simulink library "lib_transmission2"  (Simulink 4.1.1)
values from neighbouring files (symbols this model uses):
  logFlag = 1    [advSACompMaskInit.m]    (also in advSACompMaskInitR13.m)
undefined symbols (not defined in the file or in its folder): cyc_mph, fc_map_spd, fc_max_trq, fc_spd_scale, fc_trq_scale, fd_inertia, fd_loss, fd_ratio, gb_dnshift_load, gb_dnshift_spd, gb_gear_number_lookup, gb_gears_num, gb_inertia, gb_loss_const, gb_loss_input_spd_coeff, gb_loss_input_trq_coeff, gb_loss_output_spd_coeff, gb_loss_output_trq_coeff, gb_map_spd_out, gb_map_trq_in, gb_map_trq_out, gb_num_init, gb_ratio, gb_shift_delay, gb_spd_scale, gb_trq_scale, gb_upshift_load, gb_upshift_spd, htc_inertia, htc_k_adv, htc_k_adv_coast, htc_lockup, htc_lockup_load, htc_lockup_spd, htc_lu_gear_range, htc_max_coast_tr, htc_min_coast_tr, htc_pump_loss_spd, htc_pump_loss_trq_lockup, htc_pump_loss_trq_unlock, htc_sr, htc_sr_coast, htc_tr, htc_tr_coast, htc_unlock_spd, mc_map_spd, mc_max_trq, mc_overtrq_factor, mc_spd_scale, mc_trq_scale, tc_loss, tc_mc_to_fc_ratio, tx_eff_map, tx_map_spd, tx_map_trq, tx_pg_r, tx_pg_s, tx_speed_dep, vc_clutch_bool, vc_idle_spd ... (+2)
libraries: lib_controls x1, lib_etc x1, lib_controls2 x1, lib_transmission x1
(part 15 of 17)

== system lib_transmission2/hydraulic torque converter <htc> with pump loss/conventional HTC  and Interface/htc model/SR ==
  T,w req out : Inport  Port=1  LatchInput=off
  w in : Inport  Port=2  LatchInput=off
  >0 : Saturate  UpperLimit=inf  LowerLimit=eps  LinearizeAsGain=on
  Constant : Constant  Orientation=left  Value=0
  Constant1 : Constant  Value=vc_idle_spd+eps
  Constant3 : Constant  Value=1
  K_adv : Subsystem
      settings: RTWFcnNameOpts=Auto  RTWFileNameOpts=Auto
  K_adv_coast : Subsystem
      settings: RTWFcnNameOpts=Auto  RTWFileNameOpts=Auto
  Logical Operator : Logic  Operator=NOT  Inputs=1
  Logical Operator1 : Logic  Operator=NOT  Inputs=1
  MinMax : MinMax  Function=min  Inputs=2
  Relational Operator : RelationalOperator  Operator=>=
  SR Look-Up Table SR=wout/win : Lookup  InputValues=htc_k_adv  OutputValues=htc_sr
  SR Look-Up Table SR=wout/win coast : Lookup  InputValues=fliplr(htc_k_adv_coast)  OutputValues=fliplr(htc_sr_coast)
  SRmax= wout/win,min : Product  Inputs=*/  Multiplication=Element-wise(.*)  SaturateOnIntegerOverflow=on
  T : Selector  InputType=Vector  ElementSrc=Internal  Elements=1  RowSrc=Internal  Rows=1  ColumnSrc=Internal  Columns=1  InputPortWidth=2
  enhancedToWorkspace1 : Subsystem  TreatAsAtomicUnit=on  mask(enhancedToWorkspace){generalName=generalName, specificName=coasting, logFlag=logFlag}
      mask prompts: generalName "General Name [char-evaluated]"; specificName "Specific Name [char-literal]"; logFlag "Enable flag (1=on,0=off)"
      mask help: A wrapper for the Simulink "To Workspace" block that allows you to evaluate the name of the variable to log to workspace. This is useful to avoid the double logging errors that occur when you pull in two library models that attempt to log to the same variable.
      mask init:
      | enhancedToWsMaker
      settings: CopyFcn=breakLinkCopyFcn  ParentCloseFcn=breakLinkParCloseFcn  RTWFcnNameOpts=Auto  RTWFileNameOpts=Auto
      mask Help:
      | <h2>Enhanced To Workspace Block</h2>
      | <h3>Parameters</h3>
      | <UL>
      | <li><b>General Name:</b> This is the more general name of the variable. Variables are saved to the workspace as <i>generalName_specificName</i>. Note that this is an evaluated variable. If you would like to type in the value directly, it must be surrounded with single quotes. Otherwise you can input the name of a variable containing a char string.</li>
      | <li><b>Specific Name:</b> This is the specific name of the variable. Note that this is input as a char literal (i.e., you don't need quotes).</li>
      | <li><b>Enable Flag:</b> This flag should have the value of 0 or 1. If 0, the variable will not be logged to the workspace. If 1, the variable will be logged. This is done so that variable logging can be turned off to improve speed.</li>
      | </ul>
      | <h3>Overview</h3>
      | <p>The enhanced to workspace block was put together to allow one to dynamically resolve variable names at run time in simulink. This is most powerful when used in conjunction with a masked subsystem to allow multiple instances of that masked subsytem to be used in the same model. The strategy is to set the generalName in the block mask which will allow the block to change the general name for all variable logging on the fly.
      | <h3>Helper Files</h3>
      | <p>Three m-files are required by the enhancedToWorkspace block. These files are located in the &lt; ADVISOR root &gt;/GUI directory :
      | <ul>
      | <li><i>enhancedToWsMaker.m</i> This file runs the mask initialization for the block</li>
      | <li><i>breakLinkCopyFcn.m</i> This file is used by the block callback when the simulink block is copied. It is necessary to break the link to the enhancedToWorkspace similar to the To Workspace block in order for it to be able to configure itself. (Try copying simulink's To Workspace block--it is impossible to make a link)</li>
      | <li><i>breakLinkParCloseFcn.m</i> This file is similar to the breakLinkCopyFcn and is used when a parent system is closed</li>
      | </ul>
      | <hr>
      | 
      | <p>Created 2003-Jan-21, Michael Patrick O'Keefe, NREL</p>
      | 
      | <!--
      | <VARDEF>
      | <H3>var_name</H3>
      | <UL>
      | <LI><B>data type</B> data type here</LI>
      | <LI><B>units</B> units here</LI>
      | <LI><B>vehicle type</B> vehicle type here</LI>
      | <LI><B>description</B> description here</LI>
      | </UL>
      | </VARDEF>
      | -->
      mask Display: disp([generalName,'_',specificName])
  enhancedToWorkspace2 : Subsystem  TreatAsAtomicUnit=on  mask(enhancedToWorkspace){generalName=generalName, specificName=locked, logFlag=logFlag}
      mask prompts: generalName "General Name [char-evaluated]"; specificName "Specific Name [char-literal]"; logFlag "Enable flag (1=on,0=off)"
      mask help: A wrapper for the Simulink "To Workspace" block that allows you to evaluate the name of the variable to log to workspace. This is useful to avoid the double logging errors that occur when you pull in two library models that attempt to log to the same variable.
      mask init:
      | enhancedToWsMaker
      settings: CopyFcn=breakLinkCopyFcn  ParentCloseFcn=breakLinkParCloseFcn  RTWFcnNameOpts=Auto  RTWFileNameOpts=Auto
      mask Help:
      | <h2>Enhanced To Workspace Block</h2>
      | <h3>Parameters</h3>
      | <UL>
      | <li><b>General Name:</b> This is the more general name of the variable. Variables are saved to the workspace as <i>generalName_specificName</i>. Note that this is an evaluated variable. If you would like to type in the value directly, it must be surrounded with single quotes. Otherwise you can input the name of a variable containing a char string.</li>
      | <li><b>Specific Name:</b> This is the specific name of the variable. Note that this is input as a char literal (i.e., you don't need quotes).</li>
      | <li><b>Enable Flag:</b> This flag should have the value of 0 or 1. If 0, the variable will not be logged to the workspace. If 1, the variable will be logged. This is done so that variable logging can be turned off to improve speed.</li>
      | </ul>
      | <h3>Overview</h3>
      | <p>The enhanced to workspace block was put together to allow one to dynamically resolve variable names at run time in simulink. This is most powerful when used in conjunction with a masked subsystem to allow multiple instances of that masked subsytem to be used in the same model. The strategy is to set the generalName in the block mask which will allow the block to change the general name for all variable logging on the fly.
      | <h3>Helper Files</h3>
      | <p>Three m-files are required by the enhancedToWorkspace block. These files are located in the &lt; ADVISOR root &gt;/GUI directory :
      | <ul>
      | <li><i>enhancedToWsMaker.m</i> This file runs the mask initialization for the block</li>
      | <li><i>breakLinkCopyFcn.m</i> This file is used by the block callback when the simulink block is copied. It is necessary to break the link to the enhancedToWorkspace similar to the To Workspace block in order for it to be able to configure itself. (Try copying simulink's To Workspace block--it is impossible to make a link)</li>
      | <li><i>breakLinkParCloseFcn.m</i> This file is similar to the breakLinkCopyFcn and is used when a parent system is closed</li>
      | </ul>
      | <hr>
      | 
      | <p>Created 2003-Jan-21, Michael Patrick O'Keefe, NREL</p>
      | 
      | <!--
      | <VARDEF>
      | <H3>var_name</H3>
      | <UL>
      | <LI><B>data type</B> data type here</LI>
      | <LI><B>units</B> units here</LI>
      | <LI><B>vehicle type</B> vehicle type here</LI>
      | <LI><B>description</B> description here</LI>
      | </UL>
      | </VARDEF>
      | -->
      mask Display: disp([generalName,'_',specificName])
  if coasting : Switch  Threshold=eps
  "locked up, then SR=1" : Switch  Threshold=eps
  min,max : Saturate  UpperLimit=inf  LowerLimit=1  LinearizeAsGain=on
  shifting SR : Subsystem
      settings: RTWFcnNameOpts=Auto  RTWFileNameOpts=Auto
  wout,req : Selector  InputType=Vector  ElementSrc=Internal  Elements=2  RowSrc=Internal  Rows=1  ColumnSrc=Internal  Columns=1  InputPortWidth=2
  SR : Outport  Port=1  InitialOutput=0
  coasting : Outport  Port=2  InitialOutput=0
  wires:
  K_adv/1(K_adv) -> SR Look-Up Table SR=wout/win/1
  Logical Operator1/1 -> coasting/1, enhancedToWorkspace1/1(In1)
  >0/1 -> SR/1
  if coasting/1 -> >0/1
  K_adv_coast/1(K_adv_coast) -> SR Look-Up Table SR=wout/win coast/1
  MinMax/1 -> if coasting/3
  min,max/1 -> MinMax/1
  wout,req/1 -> SRmax= wout/win,min/1
  Constant1/1 -> SRmax= wout/win,min/2
  SRmax= wout/win,min/1 -> MinMax/2
  shifting SR/1(SR limited) -> if coasting/1
  "locked up, then SR=1"/1 -> shifting SR/3(SR)
  w in/1 -> shifting SR/2(w in)
  SR Look-Up Table SR=wout/win/1 -> "locked up, then SR=1"/1
  Constant3/1 -> "locked up, then SR=1"/3
  Logical Operator/1 -> "locked up, then SR=1"/2
  Relational Operator/1 -> Logical Operator1/1, if coasting/2
  T/1 -> Relational Operator/1
  Constant/1 -> Relational Operator/2
  SR Look-Up Table SR=wout/win coast/1 -> min,max/1
  T,w req out/1 -> shifting SR/1(T,w req out), K_adv/1("Req'd output trq and spd (Nm), (rad/s)"), wout,req/1, K_adv_coast/1("Req'd output trq and spd (Nm), (rad/s)"), T/1
  [locked_up] -> Logical Operator/1, enhancedToWorkspace2/1(In1)

== system lib_transmission2/hydraulic torque converter <htc> with pump loss/conventional HTC  and Interface/htc model/T, shifting ==
  TR : Inport  Port=1  LatchInput=off
  Req'd  input trq : Inport  Port=2  LatchInput=off
  Req'd output trq : Inport  Port=3  LatchInput=off
  htc_spd_in_a : Inport  Port=4  LatchInput=off
  SR : Inport  Port=5  LatchInput=off
  Memory : Memory  X0=0  InheritSampleTime=off
      settings: RTWStateStorageClass=Auto
  Memory1 : Memory  X0=0  InheritSampleTime=off
      settings: RTWStateStorageClass=Auto
  MinMax : MinMax  Function=min  Inputs=2
  TR Look-Up Table TR=Tout/Tin : Lookup  InputValues=htc_sr  OutputValues=htc_tr
  T_max : Subsystem
      settings: RTWFcnNameOpts=Auto  RTWFileNameOpts=Auto
  Tin*TR= Tout,req : Product  Inputs=2  Multiplication=Element-wise(.*)  SaturateOnIntegerOverflow=on
  engine speed estimator : Subsystem
      settings: RTWFcnNameOpts=Auto  RTWFileNameOpts=Auto
  "shifting, override zero Trequest" : Switch  Threshold=eps
  T req : Outport  Port=1
  wires:
  Tin*TR= Tout,req/1 -> Memory/1
  TR/1 -> Tin*TR= Tout,req/2
  Req'd  input trq/1 -> Tin*TR= Tout,req/1
  Memory/1 -> "shifting, override zero Trequest"/1
  T_max/1(T_max max gain from htc) -> MinMax/2
  "shifting, override zero Trequest"/1 -> MinMax/1
  TR Look-Up Table TR=Tout/Tin/1 -> T_max/2(TR)
  MinMax/1 -> T req/1
  engine speed estimator/1(Out1) -> T_max/1(w_APU)
  Memory1/1 -> TR Look-Up Table TR=Tout/Tin/1
  SR/1 -> Memory1/1
  htc_spd_in_a/1 -> engine speed estimator/1(htc_spd_in_a)
  Req'd output trq/1 -> "shifting, override zero Trequest"/3
  [shifting] -> "shifting, override zero Trequest"/2

== system lib_transmission2/hydraulic torque converter <htc> with pump loss/conventional HTC  and Interface/htc model/TR ==
  SR : Inport  Port=1  LatchInput=off
  coasting : Inport  Port=2  LatchInput=off
  1/SR*TR  for coast : Fcn  Expr=1/u
  Constant3 : Constant  Value=1
  Logical Operator : Logic  Operator=NOT  Inputs=1
  Logical Operator1 : Logic  Operator=NOT  Inputs=1
  TR Look-Up Table TR=Tout/Tin : Lookup  InputValues=htc_sr  OutputValues=htc_tr
  TR Look-Up Table TR=Tout/Tin coast : Lookup  InputValues=htc_sr_coast  OutputValues=htc_tr_coast
  effic=SR*TR : Product  Inputs=**  Multiplication=Element-wise(.*)  SaturateOnIntegerOverflow=on
  enhancedToWorkspace2 : Subsystem  TreatAsAtomicUnit=on  mask(enhancedToWorkspace){generalName=generalName, specificName=efficiency, logFlag=logFlag}
      mask prompts: generalName "General Name [char-evaluated]"; specificName "Specific Name [char-literal]"; logFlag "Enable flag (1=on,0=off)"
      mask help: A wrapper for the Simulink "To Workspace" block that allows you to evaluate the name of the variable to log to workspace. This is useful to avoid the double logging errors that occur when you pull in two library models that attempt to log to the same variable.
      mask init:
      | enhancedToWsMaker
      settings: CopyFcn=breakLinkCopyFcn  ParentCloseFcn=breakLinkParCloseFcn  RTWFcnNameOpts=Auto  RTWFileNameOpts=Auto
      mask Help:
      | <h2>Enhanced To Workspace Block</h2>
      | <h3>Parameters</h3>
      | <UL>
      | <li><b>General Name:</b> This is the more general name of the variable. Variables are saved to the workspace as <i>generalName_specificName</i>. Note that this is an evaluated variable. If you would like to type in the value directly, it must be surrounded with single quotes. Otherwise you can input the name of a variable containing a char string.</li>
      | <li><b>Specific Name:</b> This is the specific name of the variable. Note that this is input as a char literal (i.e., you don't need quotes).</li>
      | <li><b>Enable Flag:</b> This flag should have the value of 0 or 1. If 0, the variable will not be logged to the workspace. If 1, the variable will be logged. This is done so that variable logging can be turned off to improve speed.</li>
      | </ul>
      | <h3>Overview</h3>
      | <p>The enhanced to workspace block was put together to allow one to dynamically resolve variable names at run time in simulink. This is most powerful when used in conjunction with a masked subsystem to allow multiple instances of that masked subsytem to be used in the same model. The strategy is to set the generalName in the block mask which will allow the block to change the general name for all variable logging on the fly.
      | <h3>Helper Files</h3>
      | <p>Three m-files are required by the enhancedToWorkspace block. These files are located in the &lt; ADVISOR root &gt;/GUI directory :
      | <ul>
      | <li><i>enhancedToWsMaker.m</i> This file runs the mask initialization for the block</li>
      | <li><i>breakLinkCopyFcn.m</i> This file is used by the block callback when the simulink block is copied. It is necessary to break the link to the enhancedToWorkspace similar to the To Workspace block in order for it to be able to configure itself. (Try copying simulink's To Workspace block--it is impossible to make a link)</li>
      | <li><i>breakLinkParCloseFcn.m</i> This file is similar to the breakLinkCopyFcn and is used when a parent system is closed</li>
      | </ul>
      | <hr>
      | 
      | <p>Created 2003-Jan-21, Michael Patrick O'Keefe, NREL</p>
      | 
      | <!--
      | <VARDEF>
      | <H3>var_name</H3>
      | <UL>
      | <LI><B>data type</B> data type here</LI>
      | <LI><B>units</B> units here</LI>
      | <LI><B>vehicle type</B> vehicle type here</LI>
      | <LI><B>description</B> description here</LI>
      | </UL>
      | </VARDEF>
      | -->
      mask Display: disp([generalName,'_',specificName])
  if coasting : Switch  Threshold=eps
  if coasting1 : Switch  Threshold=eps
  "locked up, then TR=1" : Switch  Threshold=eps
  min,max : Saturate  UpperLimit=htc_max_coast_tr  LowerLimit=htc_min_coast_tr  LinearizeAsGain=on
  TR : Outport  Port=1  InitialOutput=0
  tag scope: htc_efficiency=scoped
  wires:
  if coasting1/1 -> [htc_efficiency], enhancedToWorkspace2/1(In1)
  1/SR*TR  for coast/1 -> if coasting1/3
  effic=SR*TR/1 -> 1/SR*TR  for coast/1, if coasting1/1
  Logical Operator1/1 -> if coasting1/2, if coasting/2
  if coasting/1 -> effic=SR*TR/2, TR/1
  coasting/1 -> Logical Operator1/1
  SR/1 -> effic=SR*TR/1, TR Look-Up Table TR=Tout/Tin/1, TR Look-Up Table TR=Tout/Tin coast/1
  min,max/1 -> if coasting/3
  TR Look-Up Table TR=Tout/Tin coast/1 -> min,max/1
  "locked up, then TR=1"/1 -> if coasting/1
  Logical Operator/1 -> "locked up, then TR=1"/2
  [locked_up] -> Logical Operator/1
  Constant3/1 -> "locked up, then TR=1"/3
  TR Look-Up Table TR=Tout/Tin/1 -> "locked up, then TR=1"/1

== system lib_transmission2/hydraulic torque converter <htc> with pump loss/conventional HTC  and Interface/htc model/effect of inertia (Nm) ==
  note: This block computes the torque required to overcome the inertia of the
      | turbine (plus 1/2 fluid in htc).
  turbine/output speed (rad/s) : Inport  Port=1  LatchInput=off
  Constant : Constant  Value=htc_inertia
  Product : Product  Inputs=2  Multiplication=Element-wise(.*)  SaturateOnIntegerOverflow=on
  d/dt : Derivative
  inertia torque (Nm) : Outport  Port=1  InitialOutput=0
  wires:
  Product/1 -> inertia torque (Nm)/1
  Constant/1 -> Product/2
  turbine/output speed (rad/s)/1 -> d/dt/1
  d/dt/1 -> Product/1

== system lib_transmission2/hydraulic torque converter <htc> with pump loss/conventional HTC  and Interface/htc model/enhancedToWorkspace ==
  In1 : Inport  Port=1  LatchInput=off
  To Workspace : ToWorkspace  VariableName=htc_trq_in_a  SampleTime=-1  SaveFormat=Array
  wires:
  In1/1 -> To Workspace/1

== system lib_transmission2/hydraulic torque converter <htc> with pump loss/conventional HTC  and Interface/htc model/enhancedToWorkspace1 ==
  In1 : Inport  Port=1  LatchInput=off
  To Workspace : ToWorkspace  VariableName=htc_spd_in_a  SampleTime=-1  SaveFormat=Array
  wires:
  In1/1 -> To Workspace/1

== system lib_transmission2/hydraulic torque converter <htc> with pump loss/conventional HTC  and Interface/htc model/enhancedToWorkspace10 ==
  In1 : Inport  Port=1  LatchInput=off
  To Workspace : ToWorkspace  VariableName=htc_spd_out_a  SampleTime=-1  SaveFormat=Array
  wires:
  In1/1 -> To Workspace/1

== system lib_transmission2/hydraulic torque converter <htc> with pump loss/conventional HTC  and Interface/htc model/enhancedToWorkspace2 ==
  In1 : Inport  Port=1  LatchInput=off
  To Workspace : ToWorkspace  VariableName=htc_trq_out_r  SampleTime=-1  SaveFormat=Array
  wires:
  In1/1 -> To Workspace/1

== system lib_transmission2/hydraulic torque converter <htc> with pump loss/conventional HTC  and Interface/htc model/enhancedToWorkspace3 ==
  In1 : Inport  Port=1  LatchInput=off
  To Workspace : ToWorkspace  VariableName=htc_spd_out_r  SampleTime=-1  SaveFormat=Array
  wires:
  In1/1 -> To Workspace/1

== system lib_transmission2/hydraulic torque converter <htc> with pump loss/conventional HTC  and Interface/htc model/enhancedToWorkspace4 ==
  In1 : Inport  Port=1  LatchInput=off
  To Workspace : ToWorkspace  VariableName=htc_sr_hist  SampleTime=-1  SaveFormat=Array
  wires:
  In1/1 -> To Workspace/1

== system lib_transmission2/hydraulic torque converter <htc> with pump loss/conventional HTC  and Interface/htc model/enhancedToWorkspace5 ==
  In1 : Inport  Port=1  LatchInput=off
  To Workspace : ToWorkspace  VariableName=htc_tr_hist  SampleTime=-1  SaveFormat=Array
  wires:
  In1/1 -> To Workspace/1

== system lib_transmission2/hydraulic torque converter <htc> with pump loss/conventional HTC  and Interface/htc model/enhancedToWorkspace6 ==
  In1 : Inport  Port=1  LatchInput=off
  To Workspace : ToWorkspace  VariableName=htc_spd_in_r  SampleTime=-1  SaveFormat=Array
  wires:
  In1/1 -> To Workspace/1

== system lib_transmission2/hydraulic torque converter <htc> with pump loss/conventional HTC  and Interface/htc model/enhancedToWorkspace7 ==
  In1 : Inport  Port=1  LatchInput=off
  To Workspace : ToWorkspace  VariableName=htc_trq_in_r  SampleTime=-1  SaveFormat=Array
  wires:
  In1/1 -> To Workspace/1

== system lib_transmission2/hydraulic torque converter <htc> with pump loss/conventional HTC  and Interface/htc model/enhancedToWorkspace8 ==
  In1 : Inport  Port=1  LatchInput=off
  To Workspace : ToWorkspace  VariableName=htc_trq_inertia  SampleTime=-1  SaveFormat=Array
  wires:
  In1/1 -> To Workspace/1

== system lib_transmission2/hydraulic torque converter <htc> with pump loss/conventional HTC  and Interface/htc model/enhancedToWorkspace9 ==
  In1 : Inport  Port=1  LatchInput=off
  To Workspace : ToWorkspace  VariableName=htc_trq_out_a  SampleTime=-1  SaveFormat=Array
  wires:
  In1/1 -> To Workspace/1

== system lib_transmission2/hydraulic torque converter <htc> with pump loss/conventional HTC  and Interface/htc model/pump loss (Nm) ==
  htc impeller speed (rad/s) : Inport  Port=1  LatchInput=off
  htc lockup signal : Inport  Port=2  LatchInput=off
  Switch : Switch  Threshold=eps
  enhancedToWorkspace6 : Subsystem  TreatAsAtomicUnit=on  mask(enhancedToWorkspace){generalName=generalName, specificName=pump_loss_trq, logFlag=logFlag}
      mask prompts: generalName "General Name [char-evaluated]"; specificName "Specific Name [char-literal]"; logFlag "Enable flag (1=on,0=off)"
      mask help: A wrapper for the Simulink "To Workspace" block that allows you to evaluate the name of the variable to log to workspace. This is useful to avoid the double logging errors that occur when you pull in two library models that attempt to log to the same variable.
      mask init:
      | enhancedToWsMaker
      settings: CopyFcn=breakLinkCopyFcn  ParentCloseFcn=breakLinkParCloseFcn  RTWFcnNameOpts=Auto  RTWFileNameOpts=Auto
      mask Help:
      | <h2>Enhanced To Workspace Block</h2>
      | <h3>Parameters</h3>
      | <UL>
      | <li><b>General Name:</b> This is the more general name of the variable. Variables are saved to the workspace as <i>generalName_specificName</i>. Note that this is an evaluated variable. If you would like to type in the value directly, it must be surrounded with single quotes. Otherwise you can input the name of a variable containing a char string.</li>
      | <li><b>Specific Name:</b> This is the specific name of the variable. Note that this is input as a char literal (i.e., you don't need quotes).</li>
      | <li><b>Enable Flag:</b> This flag should have the value of 0 or 1. If 0, the variable will not be logged to the workspace. If 1, the variable will be logged. This is done so that variable logging can be turned off to improve speed.</li>
      | </ul>
      | <h3>Overview</h3>
      | <p>The enhanced to workspace block was put together to allow one to dynamically resolve variable names at run time in simulink. This is most powerful when used in conjunction with a masked subsystem to allow multiple instances of that masked subsytem to be used in the same model. The strategy is to set the generalName in the block mask which will allow the block to change the general name for all variable logging on the fly.
      | <h3>Helper Files</h3>
      | <p>Three m-files are required by the enhancedToWorkspace block. These files are located in the &lt; ADVISOR root &gt;/GUI directory :
      | <ul>
      | <li><i>enhancedToWsMaker.m</i> This file runs the mask initialization for the block</li>
      | <li><i>breakLinkCopyFcn.m</i> This file is used by the block callback when the simulink block is copied. It is necessary to break the link to the enhancedToWorkspace similar to the To Workspace block in order for it to be able to configure itself. (Try copying simulink's To Workspace block--it is impossible to make a link)</li>
      | <li><i>breakLinkParCloseFcn.m</i> This file is similar to the breakLinkCopyFcn and is used when a parent system is closed</li>
      | </ul>
      | <hr>
      | 
      | <p>Created 2003-Jan-21, Michael Patrick O'Keefe, NREL</p>
      | 
      | <!--
      | <VARDEF>
      | <H3>var_name</H3>
      | <UL>
      | <LI><B>data type</B> data type here</LI>
      | <LI><B>units</B> units here</LI>
      | <LI><B>vehicle type</B> vehicle type here</LI>
      | <LI><B>description</B> description here</LI>
      | </UL>
      | </VARDEF>
      | -->
      mask Display: disp([generalName,'_',specificName])
  pump losses at converter mode : Lookup  InputValues=htc_pump_loss_spd  OutputValues=htc_pump_loss_trq_unlock
  pump losses at lockup mode : Lookup  InputValues=htc_pump_loss_spd  OutputValues=htc_pump_loss_trq_lockup
  pump loss  torque (Nm) : Outport  Port=1  InitialOutput=0
  wires:
  Switch/1 -> pump loss  torque (Nm)/1, enhancedToWorkspace6/1(In1)
  htc lockup signal/1 -> Switch/2
  pump losses at converter mode/1 -> Switch/3
  pump losses at lockup mode/1 -> Switch/1
  htc impeller speed (rad/s)/1 -> pump losses at lockup mode/1, pump losses at converter mode/1

== system lib_transmission2/torque coupler <tc>/tc model & interface/tc model/Block NOTES ==
  note: This block models a chain- or belt-driven torque coupler, with three gears:  one each
      | for the motor, main input (the engine or gearbox), and main output (to the gearbox
      | or final drive).  It includes losses in the chain or belt, but leaves inertia effects to be
      | considered in the appropriate component.
      |
      | The entire torque required out of the torque coupler (plus losses) is required from the
      | engine.  The engine provides only as much torque as its engine controller (see the
      | <vc> block) allows.  Any remaining unmet torque request is submitted to the motor,
      | which meets the request to the best of its ability.
      |
      | The torque converter output speed is limited by the maximum speeds of both the
      | motor and the engine.
      |
      | The loss torque is zero when the gears are not turning, and is applied at the output
      |  gear.
      |
      | The gears connecting the main input and main output to the torque converter's belt
      | or chain are assumed to be of the same size, so that main input speed = main output
  note: speed, while the motor's speed may be different.  The ratio of motor speed to main
      | output speed is stored in the variable tc_mc_to_fc_spd_ratio.

== system lib_transmission2/torque coupler <tc>/tc model & interface/tc model/enhancedToWorkspace ==
  In1 : Inport  Port=1  LatchInput=off
  Terminator : Terminator
  wires:
  In1/1 -> Terminator/1

== system lib_transmission2/torque coupler <tc>/tc model & interface/tc model/enhancedToWorkspace1 ==
  In1 : Inport  Port=1  LatchInput=off
  Terminator : Terminator
  wires:
  In1/1 -> Terminator/1

== system lib_transmission2/torque coupler <tc>/tc model & interface/tc model/enhancedToWorkspace2 ==
  In1 : Inport  Port=1  LatchInput=off
  Terminator : Terminator
  wires:
  In1/1 -> Terminator/1

== system lib_transmission2/torque coupler <tc>/tc model & interface/tc model/enhancedToWorkspace3 ==
  In1 : Inport  Port=1  LatchInput=off
  Terminator : Terminator
  wires:
  In1/1 -> Terminator/1

== system lib_transmission2/torque coupler <tc>/tc model & interface/tc model/enhancedToWorkspace4 ==
  In1 : Inport  Port=1  LatchInput=off
  Terminator : Terminator
  wires:
  In1/1 -> Terminator/1

== system lib_transmission2/torque coupler <tc>/tc model & interface/tc model/help ==

== system lib_transmission2/torque coupler <tc>/tc model & interface/tc model/loss (Nm) ==
  note: The loss torque is zero when the gears are not turning,
      | and is applied at the torque coupler's output gear.
  tc output speed (rad/s) : Inport  Port=1  LatchInput=off
  Constant : Constant  Orientation=up  Value=0
  Switch : Switch  Threshold=eps
  torque coupler loss torque (Nm) : Constant  Value=tc_loss
  drag torque (Nm) : Outport  Port=1  InitialOutput=0
  wires:
  Constant/1 -> Switch/3
  tc output speed (rad/s)/1 -> Switch/2
  Switch/1 -> drag torque (Nm)/1
  torque coupler loss torque (Nm)/1 -> Switch/1

== system lib_transmission2/torque coupler <tc> DIRECT SPLIT/tc direct split model & interface/tc direct split model/Block NOTES ==
  note: This block generically models a chain- or belt-driven torque coupler, with three gears:  one each
      | for the motor, main input (the engine or gearbox), and main output (to the gearbox
      | or final drive).  It includes losses in the chain or belt, but leaves inertia effects to be
      | considered in the appropriate component.
      |
      | The entire torque required out of the torque coupler (plus losses) is sent to the control
      | strategy. The control strategy <CS> then decides how much the electric motor
      | and the ICE must supply. It then sends the EM and ICE separate requests. The 2 sources
      | then send their achieved torque signals to the Torque Coupler, where they are added
      | and sent to the block immediately before this.
      |
      | The torque coupler output speed is limited by the maximum speeds of both the
      | motor and the engine. The loss torque is zero when the gears are not
      | turning, and is applied at the output gear.
      |
      | The gears connecting the main input and main output to the torque converter's belt
      | or chain are assumed to be of the same size, so that main input speed = main output
      | speed, while the motor's speed may be different.  The ratio of motor speed to main
      | output speed is stored in the variable tc_mc_to_fc_spd_ratio.
      |
      | NOTE: This block is modeled after the HONDA Insight. It represents a hypothetical Torque
      | Coupler, since in the Insight, the EM and ICE are on the same shaft. Change the
      | values of the ratio and inertia if modeling another torque coupler.

== system lib_transmission2/torque coupler <tc> DIRECT SPLIT/tc direct split model & interface/tc direct split model/enhancedToWorkspace ==
  In1 : Inport  Port=1  LatchInput=off
  Terminator : Terminator
  wires:
  In1/1 -> Terminator/1

== system lib_transmission2/torque coupler <tc> DIRECT SPLIT/tc direct split model & interface/tc direct split model/enhancedToWorkspace1 ==
  In1 : Inport  Port=1  LatchInput=off
  Terminator : Terminator
  wires:
  In1/1 -> Terminator/1

== system lib_transmission2/torque coupler <tc> DIRECT SPLIT/tc direct split model & interface/tc direct split model/enhancedToWorkspace2 ==
  In1 : Inport  Port=1  LatchInput=off
  Terminator : Terminator
  wires:
  In1/1 -> Terminator/1

== system lib_transmission2/torque coupler <tc> DIRECT SPLIT/tc direct split model & interface/tc direct split model/enhancedToWorkspace3 ==
  In1 : Inport  Port=1  LatchInput=off
  Terminator : Terminator
  wires:
  In1/1 -> Terminator/1

== system lib_transmission2/torque coupler <tc> DIRECT SPLIT/tc direct split model & interface/tc direct split model/enhancedToWorkspace4 ==
  In1 : Inport  Port=1  LatchInput=off
  Terminator : Terminator
  wires:
  In1/1 -> Terminator/1

== system lib_transmission2/torque coupler <tc> DIRECT SPLIT/tc direct split model & interface/tc direct split model/help ==

== system lib_transmission2/torque coupler <tc> DIRECT SPLIT/tc direct split model & interface/tc direct split model/loss (Nm) ==
  note: The loss torque is zero when the gears are not turning,
      | and is applied at the torque coupler's output gear.
      |
      | FOR THE INSIGHT, tc_loss==0
  tc output speed (rad/s) : Inport  Port=1  LatchInput=off
  Constant : Constant  Orientation=up  Value=0
  Switch : Switch  Threshold=eps
  torque coupler loss torque (Nm) : Constant  Value=tc_loss
  drag torque (Nm) : Outport  Port=1  InitialOutput=0
  wires:
  torque coupler loss torque (Nm)/1 -> Switch/1
  Switch/1 -> drag torque (Nm)/1
  tc output speed (rad/s)/1 -> Switch/2
  Constant/1 -> Switch/3

== system lib_transmission2/Clutch Control/Clutch Control/Clutch Control/clutch control/Block NOTES ==
  note: This clutch control block determines the clutch state given the req'd clutch output torque
      | and speed (labelled as gearbox input torque and speed), and the gear number history.
      |                           conditions                                                                       clutch state
      | gear is being shifted OR (trq <~ 0 AND (engine is                                     1 == disengaged
      | clutched to avoid compression braking OR spd < idle))
      |
      | (trq >~ 0) AND (spd < launch speed) AND clutch                                       2 == slipping
      | was not engaged during previous time step
      |
      | neither of above sets of conditions are met                                          3 == engaged

== system lib_transmission2/Clutch Control/Clutch Control/Clutch Control/clutch control/gearbox speed estimator ==
  gb_spd_in_r if no gear change : Inport  Port=1  LatchInput=off
  Block NOTES : Subsystem
      settings: RTWFcnNameOpts=Auto  RTWFileNameOpts=Auto
      mask Display: disp('Block\nNOTES')
  Constant : Constant  Orientation=left  Value=eps
  Constant1 : Constant  Orientation=left  Value=0
  Constant2 : Constant  Orientation=left  Value=1
  Constant3 : Constant  Orientation=left  Value=0.11
  Gain : Gain  Gain=0.447  Multiplication=Element-wise(K.*u)  SaturateOnIntegerOverflow=on
  IC : InitialCondition  Value=cyc_mph(1,2)*0.447/wh_radius*fd_ratio*gb_ratio(gb_num_init)
  IC1 : InitialCondition  Value=1
  Logical : Logic  Operator=AND  Inputs=2
  Product : Product  Inputs=**/  Multiplication=Element-wise(.*)  SaturateOnIntegerOverflow=on
  Relational : RelationalOperator  Operator=>
  Relational1 : RelationalOperator  Operator=<=
  Sum : Sum  Inputs=++  SaturateOnIntegerOverflow=on
  Sum1 : Sum  Inputs=-+  SaturateOnIntegerOverflow=on
  Switch : Switch  Threshold=eps
  Switch1 : Switch  Threshold=eps
  dt : Subsystem
      settings: RTWFcnNameOpts=Auto  RTWFileNameOpts=Auto
  Out1 : Outport  Port=1
  wires:
  dt/1(Out1) -> Relational1/1
  Logical/1 -> Switch1/2
  IC1/1 -> Logical/1
  Relational1/1 -> Logical/2
  Constant3/1 -> Relational1/2
  [gb_spd_in_a] -> Product/1
  gb_spd_in_r if no gear change/1 -> Switch1/3
  Switch1/1 -> Out1/1
  Switch/1 -> IC/1
  Relational/1 -> IC1/1
  Sum1/1 -> Relational/1
  Constant2/1 -> Relational/2
  [mpha] -> Sum1/1, Gain/1
  [cyc_mph_r] -> Sum1/2
  Constant/1 -> Sum/2
  IC/1 -> Switch1/1
  Constant1/1 -> Switch/3
  [veh_spd_a_rec] -> Switch/2, Sum/1
  Gain/1 -> Product/2
  Sum/1 -> Product/3
  Product/1 -> Switch/1

== system lib_transmission2/Gearbox Control/Gearbox Control manual shift logic/manual shift logic/gearbox  control/Block NOTES ==
  note: This gearbox control block computes the current gear number given the gearbox's
      | req'd output torque and speed and an estimate its efficiency.  Upshifts occur, given a
      | certain engine speed,  when the estimated engine load falls below the upshift curve
      | in engine speed/load space, and downshifts likewise occur when estimated engine
      | load rises above the downshift curve.  Separate upshift and downshift curves are
      | defined for each gear.  An upshift may not be immediately followed by a downshift.
      | If the tires are about to slip, don't upshift unless the engine would be at max. speed.
      | Enforce this rule by setting the load to 1 when the tires are about to slip.

== system lib_transmission2/Gearbox Control/Gearbox Control manual shift logic/manual shift logic/gearbox  control/allow downshift? ==
  prev gearnum : Inport  Port=1  LatchInput=off
  Logical Operator : Logic  Operator=NOR  Inputs=2
  Memory : Memory  X0=1  InheritSampleTime=off
      settings: RTWStateStorageClass=Auto
  Memory1 : Memory  X0=1  InheritSampleTime=off
      settings: RTWStateStorageClass=Auto
  Relational Operator1 : RelationalOperator  Operator=>
  Relational Operator2 : RelationalOperator  Operator=>
  allow shift : Outport  Port=1  InitialOutput=0
  wires:
  Logical Operator/1 -> allow shift/1
  prev gearnum/1 -> Relational Operator1/1, Memory/1, Relational Operator2/1
  Relational Operator1/1 -> Logical Operator/1
  Memory/1 -> Relational Operator1/2, Memory1/1
  Memory1/1 -> Relational Operator2/2
  Relational Operator2/1 -> Logical Operator/2

== system lib_transmission2/Gearbox Control/Gearbox Control manual shift logic/manual shift logic/gearbox  control/downshift  command ==
  prev gear number : Inport  Port=1  LatchInput=off
  engine load : Inport  Port=2  LatchInput=off
  engine speed : Inport  Port=3  LatchInput=off
  Mux : Mux  Inputs=2
      settings: DisplayOption=none
  Relational Operator : RelationalOperator  Operator=>
  load fraction : Subsystem  mask(Gear Selector){spd=gb_dnshift_spd, load=gb_dnshift_load}
      mask prompts: spd "Speeds:"; load "Load Fractions:"
      mask help:
      | This block will perform a linear interplation (extrapolation outside of bounds) to determine the shift point load fraction associated with the current gear number and speed.
      |
      | The Speeds parameter should be defined as an array of vectors containing speeds for each gear number.  The Load Fractions parameter should be defined as a array of vectors containing load fractions indexed by the speeds in the Speeds parameter for each gear number.
      settings: RTWFcnNameOpts=Auto  RTWFileNameOpts=Auto
      mask Help:
      | Reference the base workspace variables - gb_**shift_spd and gb_**shift_load  where ** is either up for upshift conditions or dn for downshift conditions.
      | 
      | Or define the arrays as follows:
      | 
      | {[spd1 spd2 spd3 spd4]; [spd1 spd2 spd3 spd4]; ...}
      | 
      | {[load1 load2 load3 load4]; [load1 load2 load3 load4]; ...}
      | 
      | where each array contains one row for each gear in the gearbox.  Speeds should be defined in rad/s and loads as a decimal fraction.
  command : Outport  Port=1  InitialOutput=0
  wires:
  load fraction/1(Out1) -> Relational Operator/2
  Mux/1 -> load fraction/1(In1)
  engine load/1 -> Relational Operator/1
  prev gear number/1 -> Mux/1
  engine speed/1 -> Mux/2
  Relational Operator/1 -> command/1

== system lib_transmission2/Gearbox Control/Gearbox Control manual shift logic/manual shift logic/gearbox  control/gearbox speed estimator ==
  gb_spd_in_r if no gear change : Inport  Port=1  LatchInput=off
  Block NOTES : Subsystem
      settings: RTWFcnNameOpts=Auto  RTWFileNameOpts=Auto
      mask Display: disp('Block\nNOTES')
  Constant : Constant  Orientation=left  Value=eps
  Constant1 : Constant  Orientation=left  Value=0
  Constant2 : Constant  Orientation=left  Value=1
  Constant3 : Constant  Orientation=left  Value=0.11
  Gain : Gain  Gain=0.447  Multiplication=Element-wise(K.*u)  SaturateOnIntegerOverflow=on
  IC : InitialCondition  Value=cyc_mph(1,2)*0.447/wh_radius*fd_ratio*gb_ratio(gb_num_init)
  IC1 : InitialCondition  Value=1
  Logical : Logic  Operator=AND  Inputs=2
  Product : Product  Inputs=**/  Multiplication=Element-wise(.*)  SaturateOnIntegerOverflow=on
  Relational : RelationalOperator  Operator=>
  Relational1 : RelationalOperator  Operator=<=
  Sum : Sum  Inputs=++  SaturateOnIntegerOverflow=on
  Sum1 : Sum  Inputs=-+  SaturateOnIntegerOverflow=on
  Switch : Switch  Threshold=eps
  Switch1 : Switch  Threshold=eps
  dt : Subsystem
      settings: RTWFcnNameOpts=Auto  RTWFileNameOpts=Auto
  Out1 : Outport  Port=1
  wires:
  Product/1 -> Switch/1
  Sum/1 -> Product/3
  Gain/1 -> Product/2
  [veh_spd_a_rec] -> Sum/1, Switch/2
  Constant1/1 -> Switch/3
  IC/1 -> Switch1/1
  Constant/1 -> Sum/2
  [cyc_mph_r] -> Sum1/2
  [mpha] -> Gain/1, Sum1/1
  Constant2/1 -> Relational/2
  Sum1/1 -> Relational/1
  Relational/1 -> IC1/1
  Switch/1 -> IC/1
  Switch1/1 -> Out1/1
  gb_spd_in_r if no gear change/1 -> Switch1/3
  [gb_spd_in_a] -> Product/1
  Constant3/1 -> Relational1/2
  Relational1/1 -> Logical/2
  IC1/1 -> Logical/1
  Logical/1 -> Switch1/2
  dt/1(Out1) -> Relational1/1

== system lib_transmission2/Gearbox Control/Gearbox Control manual shift logic/manual shift logic/gearbox  control/shifting1 ==
  gear number : Inport  Port=1  LatchInput=off
  Constant : Constant  Value=gb_shift_delay-1e-6
  Relational Operator : RelationalOperator  Operator=<
  time since last shift : Subsystem
      settings: RTWFcnNameOpts=Auto  RTWFileNameOpts=Auto
      mask Display: disp('time since\nlast shift')
  out_1 : Outport  Port=1  InitialOutput=0
  wires:
  Relational Operator/1 -> out_1/1
  gear number/1 -> time since last shift/1(in_1)
  Constant/1 -> Relational Operator/2
  time since last shift/1(out_1) -> Relational Operator/1

== system lib_transmission2/Gearbox Control/Gearbox Control manual shift logic/manual shift logic/gearbox  control/upshift  command ==
  prev gear number : Inport  Port=1  LatchInput=off
  engine load : Inport  Port=2  LatchInput=off
  engine speed : Inport  Port=3  LatchInput=off
  Mux : Mux  Inputs=2
      settings: DisplayOption=none
  Relational Operator : RelationalOperator  Operator=<
  load fraction : Subsystem  mask(Gear Selector){spd=gb_upshift_spd, load=gb_upshift_load}
      mask prompts: spd "Speeds:"; load "Load Fractions:"
      mask help:
      | This block will perform a linear interplation (extrapolation outside of bounds) to determine the shift point load fraction associated with the current gear number and speed.
      |
      | The Speeds parameter should be defined as an array of vectors containing speeds for each gear number.  The Load Fractions parameter should be defined as a array of vectors containing load fractions indexed by the speeds in the Speeds parameter for each gear number.
      settings: RTWFcnNameOpts=Auto  RTWFileNameOpts=Auto
      mask Help:
      | Reference the base workspace variables - gb_**shift_spd and gb_**shift_load  where ** is either up for upshift conditions or dn for downshift conditions.
      | 
      | Or define the arrays as follows:
      | 
      | {[spd1 spd2 spd3 spd4]; [spd1 spd2 spd3 spd4]; ...}
      | 
      | {[load1 load2 load3 load4]; [load1 load2 load3 load4]; ...}
      | 
      | where each array contains one row for each gear in the gearbox.  Speeds should be defined in rad/s and loads as a decimal fraction.
  command : Outport  Port=1  InitialOutput=0
  wires:
  load fraction/1(Out1) -> Relational Operator/2
  engine load/1 -> Relational Operator/1
  prev gear number/1 -> Mux/1
  Mux/1 -> load fraction/1(In1)
  engine speed/1 -> Mux/2
  Relational Operator/1 -> command/1

== system lib_transmission2/Gearbox Control/automatic transmission gearbox and htc advanced lock-up logic for htc shift logic for gearbox/gearbox control for use w/ AT/Speed Dependent Shifting/shifting ==
  gear number : Inport  Port=1  LatchInput=off
  Constant : Constant  Value=gb_shift_delay-1e-6
  Relational Operator : RelationalOperator  Operator=<
  time since last shift : Subsystem
      settings: RTWFcnNameOpts=Auto  RTWFileNameOpts=Auto
      mask Display: disp('time since\nlast shift')
  out_1 : Outport  Port=1  InitialOutput=0
  wires:
  time since last shift/1(out_1) -> Relational Operator/1
  Constant/1 -> Relational Operator/2
  gear number/1 -> time since last shift/1(in_1)
  Relational Operator/1 -> out_1/1

== system lib_transmission2/Gearbox Control/automatic transmission gearbox and htc advanced lock-up logic for htc shift logic for gearbox/gearbox control for use w/ AT/Speed Dependent Shifting/shifting1 ==
  gear number : Inport  Port=1  LatchInput=off
  Constant : Constant  Value=gb_shift_delay-1e-6
  Relational Operator : RelationalOperator  Operator=<
  time since last shift : Subsystem
      settings: RTWFcnNameOpts=Auto  RTWFileNameOpts=Auto
      mask Display: disp('time since\nlast shift')
  out_1 : Outport  Port=1  InitialOutput=0
  wires:
  time since last shift/1(out_1) -> Relational Operator/1
  Constant/1 -> Relational Operator/2
  gear number/1 -> time since last shift/1(in_1)
  Relational Operator/1 -> out_1/1

== system lib_transmission2/Gearbox Control/automatic transmission gearbox and htc advanced lock-up logic for htc shift logic for gearbox/gearbox control for use w/ AT/downshift  command/load fraction ==
  In1 : Inport  Port=1  LatchInput=off
  S-Function : S-Function  FunctionName=sfun_gearbox  Parameters=load, spd  PortCounts=[]  SFunctionModules=''
  Out1 : Outport  Port=1  InitialOutput=0
  wires:
  S-Function/1 -> Out1/1
  In1/1 -> S-Function/1

== system lib_transmission2/Gearbox Control/automatic transmission gearbox and htc advanced lock-up logic for htc shift logic for gearbox/gearbox control for use w/ AT/downshift  command1/load fraction ==
  In1 : Inport  Port=1  LatchInput=off
  S-Function : S-Function  FunctionName=sfun_gearbox  Parameters=load, spd  PortCounts=[]  SFunctionModules=''
  Out1 : Outport  Port=1  InitialOutput=0
  wires:
  In1/1 -> S-Function/1
  S-Function/1 -> Out1/1

== system lib_transmission2/Gearbox Control/automatic transmission gearbox and htc advanced lock-up logic for htc shift logic for gearbox/gearbox control for use w/ AT/est. engine trq and spd/Block NOTES ==
  note: Estimate engine torque and speed associated with the previous gear, assuming that
      | the gearbox efficiency is constant.

== system lib_transmission2/Gearbox Control/automatic transmission gearbox and htc advanced lock-up logic for htc shift logic for gearbox/gearbox control for use w/ AT/est. engine trq and spd/K_adv ==
  "Req'd output trq and spd (Nm), (rad/s)" : Inport  Port=1  LatchInput=off
  K_adv=wout/(Tout)^0.5 : Fcn  Expr=u[2]/u[1]^0.5
  Saturation : Saturate  UpperLimit=max(htc_k_adv)  LowerLimit=min(htc_k_adv)  LinearizeAsGain=on
  Saturation2 : Saturate  UpperLimit=inf  LowerLimit=eps  LinearizeAsGain=on
  K_adv : Outport  Port=1
  wires:
  "Req'd output trq and spd (Nm), (rad/s)"/1 -> Saturation2/1
  Saturation2/1 -> K_adv=wout/(Tout)^0.5/1
  K_adv=wout/(Tout)^0.5/1 -> Saturation/1
  Saturation/1 -> K_adv/1

== system lib_transmission2/Gearbox Control/automatic transmission gearbox and htc advanced lock-up logic for htc shift logic for gearbox/gearbox control for use w/ AT/est. engine trq and spd assuming lockup/Block NOTES ==
  note: Estimate engine torque and speed associated with the current gear, assuming that
      | the gearbox efficiency is constant.

== system lib_transmission2/Gearbox Control/automatic transmission gearbox and htc advanced lock-up logic for htc shift logic for gearbox/gearbox control for use w/ AT/shifting1/time since last shift ==
  in_1 : Inport  Port=1  LatchInput=off
  just shifted : Subsystem
      settings: RTWFcnNameOpts=Auto  RTWFileNameOpts=Auto
      mask Display: disp('just\nshifted')
  timer : Subsystem
      settings: RTWFcnNameOpts=Auto  RTWFileNameOpts=Auto
      mask Display: disp('timer')
  out_1 : Outport  Port=1  InitialOutput=0
  wires:
  in_1/1 -> just shifted/1(in_1)
  just shifted/1(out_1) -> timer/1(trigger)
  timer/1(time) -> out_1/1

== system lib_transmission2/Gearbox Control/automatic transmission gearbox and htc advanced lock-up logic for htc shift logic for gearbox/gearbox control for use w/ AT/upshift  command/load fraction ==
  In1 : Inport  Port=1  LatchInput=off
  S-Function : S-Function  FunctionName=sfun_gearbox  Parameters=load, spd  PortCounts=[]  SFunctionModules=''
  Out1 : Outport  Port=1  InitialOutput=0
  wires:
  S-Function/1 -> Out1/1
  In1/1 -> S-Function/1

== system lib_transmission2/Gearbox Control/automatic transmission gearbox and htc standard lockup logic for htc shift logic for gearbox/gearbox control for use w/ AT/downshift  command/load fraction ==
  In1 : Inport  Port=1  LatchInput=off
  S-Function : S-Function  FunctionName=sfun_gearbox  Parameters=load, spd  PortCounts=[]  SFunctionModules=''
  Out1 : Outport  Port=1  InitialOutput=0
  wires:
  In1/1 -> S-Function/1
  S-Function/1 -> Out1/1

== system lib_transmission2/Gearbox Control/automatic transmission gearbox and htc standard lockup logic for htc shift logic for gearbox/gearbox control for use w/ AT/downshift  command1/load fraction ==
  In1 : Inport  Port=1  LatchInput=off
  S-Function : S-Function  FunctionName=sfun_gearbox  Parameters=load, spd  PortCounts=[]  SFunctionModules=''
  Out1 : Outport  Port=1  InitialOutput=0
  wires:
  S-Function/1 -> Out1/1
  In1/1 -> S-Function/1

== system lib_transmission2/Gearbox Control/automatic transmission gearbox and htc standard lockup logic for htc shift logic for gearbox/gearbox control for use w/ AT/est. engine trq and spd/Block NOTES ==
  note: Estimate engine torque and speed associated with the previous gear, assuming that
      | the gearbox efficiency is constant.

== system lib_transmission2/Gearbox Control/automatic transmission gearbox and htc standard lockup logic for htc shift logic for gearbox/gearbox control for use w/ AT/est. engine trq and spd/K_adv ==
  "Req'd output trq and spd (Nm), (rad/s)" : Inport  Port=1  LatchInput=off
  K_adv=wout/(Tout)^0.5 : Fcn  Expr=u[2]/u[1]^0.5
  Saturation : Saturate  UpperLimit=max(htc_k_adv)  LowerLimit=min(htc_k_adv)  LinearizeAsGain=on
  Saturation2 : Saturate  UpperLimit=inf  LowerLimit=eps  LinearizeAsGain=on
  K_adv : Outport  Port=1
  wires:
  Saturation/1 -> K_adv/1
  K_adv=wout/(Tout)^0.5/1 -> Saturation/1
  Saturation2/1 -> K_adv=wout/(Tout)^0.5/1
  "Req'd output trq and spd (Nm), (rad/s)"/1 -> Saturation2/1

== system lib_transmission2/Gearbox Control/automatic transmission gearbox and htc standard lockup logic for htc shift logic for gearbox/gearbox control for use w/ AT/est. engine trq and spd assuming lockup/Block NOTES ==
  note: Estimate engine torque and speed associated with the current gear, assuming that
      | the gearbox efficiency is constant.
